simulink model "Problem1_6"  (R2018a)
settings: Solver=VariableStepAuto  StartTime=0.0  StopTime=10  RelTol=1e-3
settings Model: Creator=NIMA  LastModifiedBy=NIMA

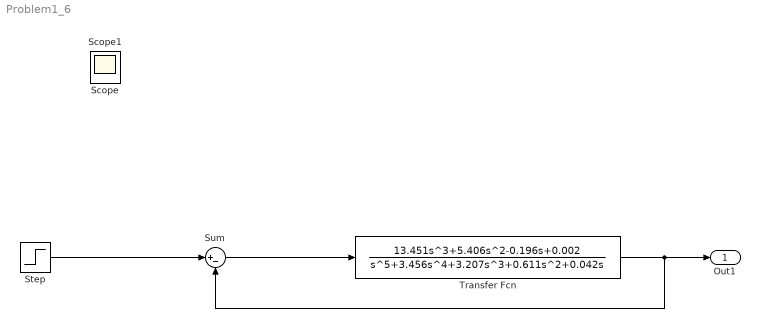
== system Problem1_6 ==
  Step : Step  SampleTime=0
  Sum : Sum  Inputs=|+-
  Transfer Fcn : TransferFcn  Numerator=[13.451 5.406 -0.196 0.002]  Denominator=[1 3.456 3.207 0.611 0.042 0]
  Out1 : Outport
  Scope : Scope
  Scope1 : Scope
  wires:
  Transfer Fcn/1 -> Sum/2, Out1/1
  Sum/1 -> Transfer Fcn/1
  Step/1 -> Sum/1
